simulink model "ex2a"  (R2020a)
settings: Solver=VariableStepAuto  StartTime=0.0  StopTime=100  RelTol=1e-3
settings Model: Creator=mumun  LastModifiedBy=mumun

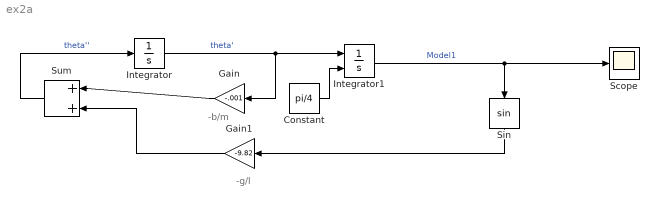
== system ex2a ==
  note: -g/l
  note: -b/m
  Constant : Constant  Value=pi/4
  Gain : Gain  Gain=-.001
  Gain1 : Gain  Gain=-9.82
  Integrator : Integrator
  Integrator1 : Integrator  InitialConditionSource=external
  Scope : Scope
  Sin : Trigonometry
  Sum : Sum  Inputs=|++
  wires:
  Integrator/1 -> Gain/1, Integrator1/1  "theta'"
  Integrator1/1 -> Scope/1, Sin/1  "Model1"
  Sin/1 -> Gain1/1
  Gain/1 -> Sum/1
  Gain1/1 -> Sum/2
  Sum/1 -> Integrator/1  "theta''"
  Constant/1 -> Integrator1/2
